simulink model "hdd_notch_final_2"  (R2015b)
settings: Solver=VariableStepAuto  StartTime=0.0  StopTime=7.0  RelTol=1e-3
undefined symbols (not defined in the file or in its folder): DiscIntNeverNeededParam
settings Model: disc_configurable_lib=simulink_discrete_with_notch_disc_lib  Creator=mac  LastModifiedBy=mac

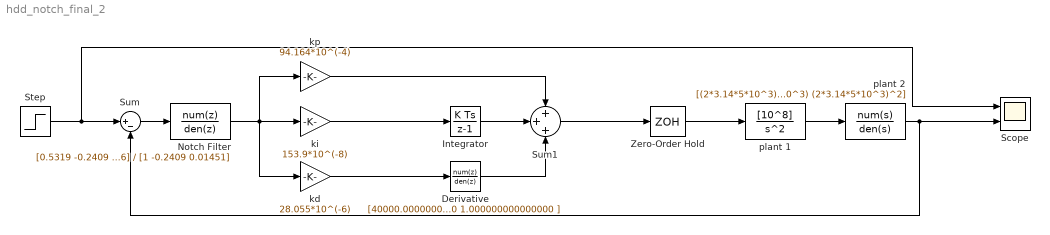
== system hdd_notch_final_2 ==
  " plant 1" : TransferFcn  Numerator=[10^8]  Denominator=[1 0 0]
  Derivative : DiscreteTransferFcn  Numerator=[40000.000000000000000 -40000.000000000000000 ]  Denominator=[1.000000000000000 1.000000000000000 ]  SampleTime=5.00000000000000024e-05
  Integrator : DiscreteIntegrator  SampleTime=5.00000000000000024e-05  ICPrevOutput=DiscIntNeverNeededParam  ICPrevScaledInput=DiscIntNeverNeededParam  mask(DiscretizedDiscreteIntegrator){}
      mask init:
      | %zoh
  Notch Filter : DiscreteTransferFcn  Numerator=[0.5319 -0.2409 0.4826]  Denominator=[1 -0.2409 0.01451]  SampleTime=5e-05
  Scope : Scope  NumInputPorts=2
  Step : Step  SampleTime=5.00000000000000024e-05  mask(DiscretizedSource){}
      mask init:
      | %zoh
  Sum : Sum  Inputs=|+-
  Sum1 : Sum  Inputs=+++
  Zero-Order Hold : ZeroOrderHold  SampleTime=5e-05
  kd : Gain  Gain=28.055*10^(-6)
  ki : Gain  Gain=153.9*10^(-8)
  kp : Gain  Gain=94.164*10^(-4)
  plant 2 : TransferFcn  Numerator=[(2*3.14*5*10^3)^2]  Denominator="[1  2*0.05*(2*3.14*5*10^3) (2*3.14*5*10^3)^2]"
  wires:
  Zero-Order Hold/1 -> " plant 1"/1
  Sum1/1 -> Zero-Order Hold/1
  Integrator/1 -> Sum1/2
  ki/1 -> Integrator/1
  kd/1 -> Derivative/1
  Derivative/1 -> Sum1/3
  kp/1 -> Sum1/1
  Sum/1 -> Notch Filter/1
  Notch Filter/1 -> kp/1, kd/1, ki/1
  Step/1 -> Scope/1, Sum/1
  " plant 1"/1 -> plant 2/1
  plant 2/1 -> Scope/2, Sum/2
